simulink model "Iteration_2"  (R2025b)
settings: Solver=ode45  StartTime=0.0  StopTime=t_end  RelTol=1e-3
values from neighbouring files (symbols this model uses):
  A = [ -(Cf + Cr)/(m*vx),            ((lr*Cr - lf*Cf)/(m*vx)) - vx,   0,   0 ... (first row only)    [Init_Script.m]    (also in lka_phase3_results.mat = [0  20; 0  0])
  B = [ Cf/m ... (first row only)    [Init_Script.m]    (also in lka_phase3_results.mat = [0 7.40740740741])
  C = [ 0, 0, 1, 0 ... (first row only)    [Init_Script.m]
  D = [ 0 ... (first row only)    [Init_Script.m]
  K = [10 8]    [lka_phase3_results.mat]
  v = 20    [lka_phase3_results.mat]
  x0 = [0; 0; 0.3; 0.05]    [Init_Script.m]    (also in lka_phase3_results.mat = [0.3 0.05])
undefined symbols (not defined in the file or in its folder): B_aug, D_aug
settings Model: Creator=Ayan  LastModifiedBy=Ayan

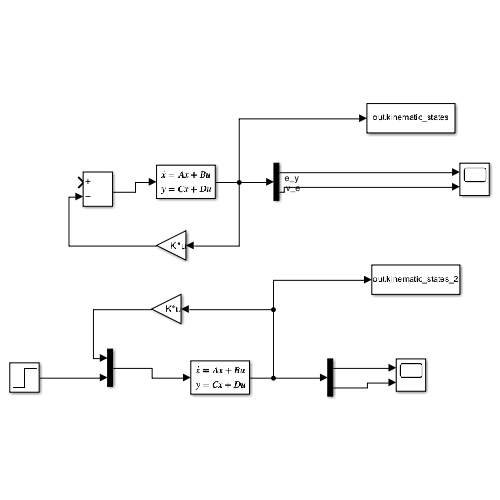
[thumbnail: Simulink's stored preview of the top-level diagram]
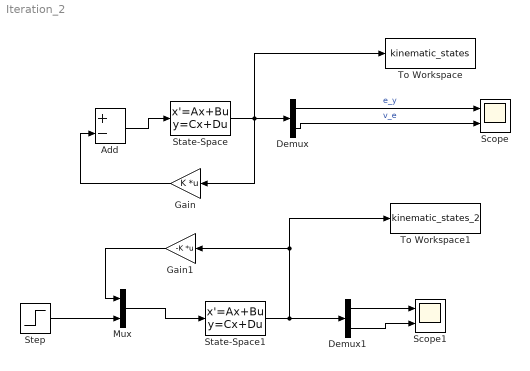
== system Iteration_2 ==
  Add : Sum  Inputs=+-
  Demux : Demux  Outputs=2
  Demux1 : Demux  Outputs=2
  Gain : Gain  Gain=K  Multiplication=Matrix(K*u)
  Gain1 : Gain  Gain=-K  Multiplication=Matrix(K*u)
  Mux : Mux  Inputs=2
  Scope : Scope  NumInputPorts=2
      settings: ActiveDisplayYMinimum=-0.32044456505002927  ActiveDisplayYMaximum=0.37006519352721345
  Scope1 : Scope  NumInputPorts=2
      settings: ActiveDisplayYMinimum=-0.00062145422426774578  ActiveDisplayYMaximum=8.016769961972418E-5
  State-Space : StateSpace  A=A  B=B  C=C  D=D  InitialCondition=x0
  State-Space1 : StateSpace  A=A  B=B_aug  C=C  D=D_aug  InitialCondition=[0, 0]
  Step : Step  After=v / 500  SampleTime=0
  To Workspace : ToWorkspace  VariableName=kinematic_states  SaveFormat=Timeseries  SampleTime=-1
  To Workspace1 : ToWorkspace  VariableName=kinematic_states_2  SaveFormat=Timeseries  SampleTime=-1
  wires:
  Add/1 -> State-Space/1
  State-Space/1 -> To Workspace/1, Gain/1, Demux/1
  Gain/1 -> Add/2
  Demux/1 -> Scope/1  "e_y"
  Demux/2 -> Scope/2  "v_e"
  Mux/1 -> State-Space1/1
  Step/1 -> Mux/2
  State-Space1/1 -> To Workspace1/1, Gain1/1, Demux1/1
  Gain1/1 -> Mux/1
  Demux1/1 -> Scope1/1
  Demux1/2 -> Scope1/2
